simulink model "IFAC20_Random_Exp1_Switched"  (R2019a)
settings: Solver=ode45  StartTime=0.0  StopTime=30  FixedStep=0.05  MaxStep=0.06  RelTol=1e-3  EnableMultiTasking=on
model workspace (MAT data in the model file):
  MCOS : class17 (value not decoded)
values from neighbouring files (symbols this model uses):
  motor_trigger = 1.1    [IFAC20_Experiment2.m]    (also in IFAC20_Experiment3.m = 0.9; IFAC20_Experiment4.m = 0.9)
  wind_trigger = 0.9    [IFAC20_Experiment2.m]    (also in IFAC20_Experiment3.m; IFAC20_Experiment4.m)
undefined symbols (not defined in the file or in its folder): altitude_error, Continuous, IC, quadModel, RPM1, RPM2, RPM3, RPM4, Time
libraries: simulink x9, ctrlSharedLib x4
(part 2 of 2)

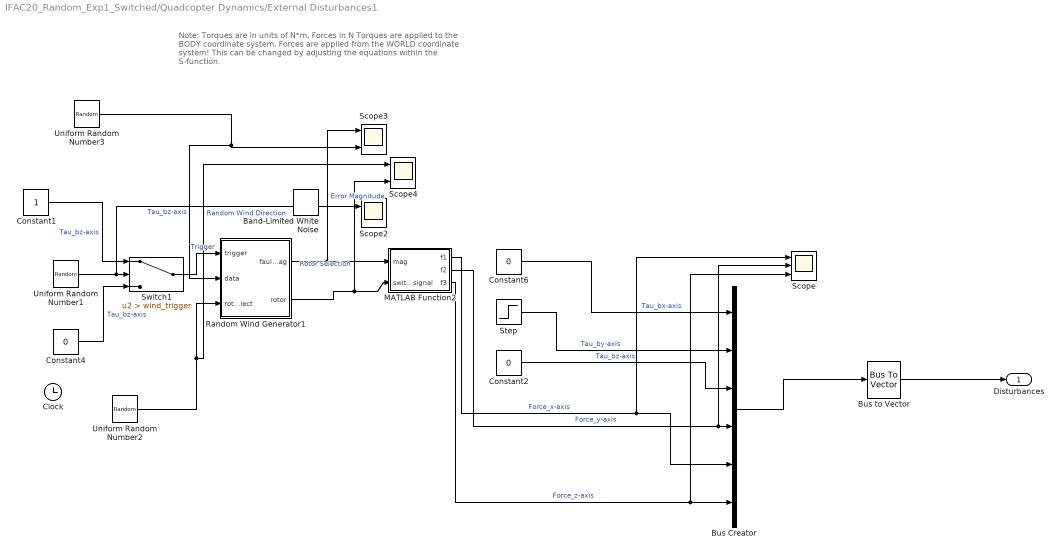
== system IFAC20_Random_Exp1_Switched/Quadcopter Dynamics/External Disturbances1 ==
  note: Note: Torques are in units of N*m, Forces in N
      | Torques are applied to the BODY coordinate system.
      | Forces are applied from the WORLD coordinate system!
      | This can be changed by adjusting the equations within the S-function.
  Band-Limited White Noise : simulink/Sources/Band-Limited White Noise  Cov=[0]  Ts=0.3  seed=[23341]
  Bus Creator : BusCreator  Inputs=6
  Bus to Vector : BusToVector
  Clock : Clock
  Constant1 : Constant
  Constant2 : Constant  Value=0
  Constant4 : Constant  Value=0
  Constant6 : Constant  Value=0
  MATLAB Function2 : MATLAB Function  TreatAsAtomicUnit=on
  Random Wind Generator1 : MATLAB Function  TreatAsAtomicUnit=on
  Scope : Scope  NumInputPorts=3
  Scope2 : Scope  NumInputPorts=2
  Scope3 : Scope  NumInputPorts=2
  Scope4 : Scope  NumInputPorts=2
  Step : Step  After=0  SampleTime=0
  Switch1 : Switch  Criteria=u2 > Threshold  Threshold=wind_trigger
  Uniform Random Number1 : UniformRandomNumber  Minimum=0  Seed=floor(rand(1)*100)  SampleTime=0.1
  Uniform Random Number2 : UniformRandomNumber  Minimum=0.5  Maximum=3.5  Seed=floor(rand(1)*100)  SampleTime=0.1
  Uniform Random Number3 : UniformRandomNumber  Minimum=0  Maximum=10  Seed=floor(rand(1)*100)  SampleTime=0.1
  "Disturbances " : Outport
  wires:
  MATLAB Function2/2(f2) -> Scope/2, Bus Creator/4  "Force_y-axis"
  Random Wind Generator1/1(fault_mag) -> Scope3/1, MATLAB Function2/1(mag)  "Error Magnitude"
  Bus Creator/1 -> Bus to Vector/1
  Constant1/1 -> Switch1/1  "Tau_bz-axis"
  Constant4/1 -> Switch1/3  "Tau_bz-axis"
  Switch1/1 -> Random Wind Generator1/1(trigger)  "Trigger"
  Uniform Random Number3/1 -> Random Wind Generator1/2(data), Scope3/2  "Tau_bz-axis"
  Constant6/1 -> Bus Creator/1  "Tau_bx-axis"
  Bus to Vector/1 -> "Disturbances "/1
  Uniform Random Number1/1 -> Scope2/1, Switch1/2
  Uniform Random Number2/1 -> Scope4/1, Random Wind Generator1/3(rotor_select)  "Random Wind Direction"
  Step/1 -> Bus Creator/2  "Tau_by-axis"
  MATLAB Function2/1(f1) -> Scope/1, Bus Creator/5  "Force_x-axis"
  Random Wind Generator1/2(rotor) -> Scope4/2, MATLAB Function2/2(switch_signal)  "Rotor Selection"
  Constant2/1 -> Bus Creator/3  "Tau_bz-axis"
  MATLAB Function2/3(f3) -> Scope/3, Bus Creator/6  "Force_z-axis"

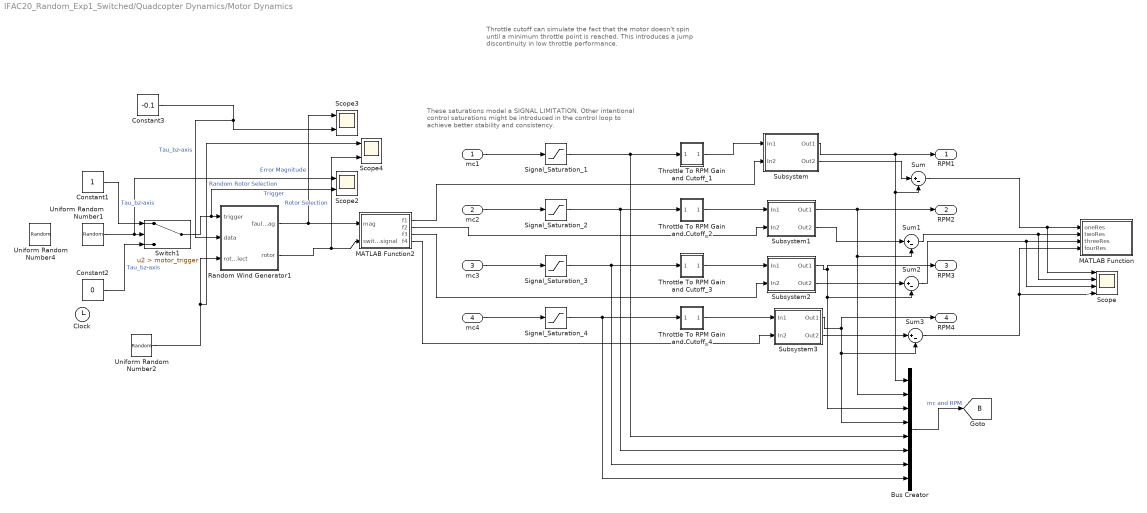
== system IFAC20_Random_Exp1_Switched/Quadcopter Dynamics/Motor Dynamics ==
  note: Throttle cutoff can simulate the fact that the motor doesn't
      | spin until a minimum throttle point is reached. This introduces
      | a jump discontinuity in low throttle performance.
  note: These saturations model a SIGNAL LIMITATION.
      | Other intentional control saturations might be introduced in the
      | control loop to achieve better stability and consistency.
  mc1 : Inport
  mc2 : Inport  Port=2
  mc3 : Inport  Port=3
  mc4 : Inport  Port=4
  Bus Creator : BusCreator  Inputs=8
  Clock : Clock
  Constant1 : Constant
  Constant2 : Constant  Value=0
  Constant3 : Constant  Value=-0.1
  MATLAB Function : MATLAB Function  TreatAsAtomicUnit=on
  MATLAB Function2 : MATLAB Function  TreatAsAtomicUnit=on
  Random Wind Generator1 : MATLAB Function  TreatAsAtomicUnit=on
  Scope : Scope  NumInputPorts=4
  Scope2 : Scope  NumInputPorts=2
  Scope3 : Scope  NumInputPorts=2
  Scope4 : Scope  NumInputPorts=2
  Signal_Saturation_{1..4} (4 alike) : Saturate  UpperLimit=100  LowerLimit=0
  Subsystem : Subsystem
  Subsystem1 : Subsystem
  Subsystem2 : Subsystem
  Subsystem3 : Subsystem
  Sum{,1..3} (4 alike) : Sum  Inputs=|+-
  Switch1 : Switch  Criteria=u2 > Threshold  Threshold=motor_trigger
  Throttle To RPM Gain and Cutoff_1 : Subsystem
  Throttle To RPM Gain and Cutoff_2 : Subsystem
  Throttle To RPM Gain and Cutoff_3 : Subsystem
  Throttle To RPM Gain and Cutoff_4 : Subsystem
  Uniform Random Number1 : UniformRandomNumber  Minimum=0  Seed=floor(rand(1)*100)  SampleTime=0.1
  Uniform Random Number2 : UniformRandomNumber  Minimum=0.5  Maximum=4.5  Seed=floor(rand(1)*100)  SampleTime=0.1
  Uniform Random Number4 : UniformRandomNumber  Minimum=0  Seed=floor(rand(1)*100)  SampleTime=0.1
  RPM1 : Outport
  RPM2 : Outport  Port=2
  RPM3 : Outport  Port=3
  RPM4 : Outport  Port=4
  tag scope: B=global
  wires:
  mc1/1 -> Signal_Saturation_1/1
  mc4/1 -> Signal_Saturation_4/1
  mc2/1 -> Signal_Saturation_2/1
  mc3/1 -> Signal_Saturation_3/1
  Signal_Saturation_1/1 -> Bus Creator/5, Throttle To RPM Gain and Cutoff_1/1(In5)
  Signal_Saturation_2/1 -> Bus Creator/6, Throttle To RPM Gain and Cutoff_2/1(In5)
  Signal_Saturation_3/1 -> Bus Creator/7, Throttle To RPM Gain and Cutoff_3/1(In5)
  Signal_Saturation_4/1 -> Bus Creator/8, Throttle To RPM Gain and Cutoff_4/1(In5)
  Throttle To RPM Gain and Cutoff_4/1(Out5) -> Subsystem3/1(In1)
  Subsystem3/1(Out1) -> RPM4/1, Sum3/2, Bus Creator/4
  Bus Creator/1 -> [B]  "mc and RPM"
  Subsystem/1(Out1) -> Sum/2, Bus Creator/1, RPM1/1
  Throttle To RPM Gain and Cutoff_1/1(Out5) -> Subsystem/1(In1)
  MATLAB Function2/1(f1) -> Subsystem/2(In2)
  Subsystem2/1(Out1) -> Sum2/2, Bus Creator/3, RPM3/1
  Subsystem1/1(Out1) -> Sum1/2, Bus Creator/2, RPM2/1
  Throttle To RPM Gain and Cutoff_2/1(Out5) -> Subsystem1/1(In1)
  Throttle To RPM Gain and Cutoff_3/1(Out5) -> Subsystem2/1(In1)
  MATLAB Function2/3(f3) -> Subsystem2/2(In2)
  MATLAB Function2/4(f4) -> Subsystem3/2(In2)
  MATLAB Function2/2(f2) -> Subsystem1/2(In2)
  Subsystem/2(Out2) -> Sum/1
  Sum/1 -> Scope/1, MATLAB Function/1(oneRes)
  Subsystem3/2(Out2) -> Sum3/1
  Subsystem2/2(Out2) -> Sum2/1
  Subsystem1/2(Out2) -> Sum1/1
  Sum3/1 -> Scope/4, MATLAB Function/4(fourRes)
  Sum2/1 -> Scope/3, MATLAB Function/3(threeRes)
  Sum1/1 -> Scope/2, MATLAB Function/2(twoRes)
  Random Wind Generator1/1(fault_mag) -> Scope3/1, MATLAB Function2/1(mag)  "Error Magnitude"
  Constant2/1 -> Switch1/3  "Tau_bz-axis"
  Uniform Random Number2/1 -> Scope4/1, Random Wind Generator1/3(rotor_select)  "Random Rotor Selection"
  Random Wind Generator1/2(rotor) -> Scope4/2, MATLAB Function2/2(switch_signal)  "Rotor Selection"
  Uniform Random Number1/1 -> Scope2/1, Switch1/2
  Constant1/1 -> Switch1/1  "Tau_bz-axis"
  Constant3/1 -> Random Wind Generator1/2(data), Scope3/2  "Tau_bz-axis"
  Switch1/1 -> Scope2/2, Random Wind Generator1/1(trigger)  "Trigger"

== system IFAC20_Random_Exp1_Switched/Quadcopter Dynamics/Motor Dynamics/Subsystem ==
  note: kalman filter
  note: Multiplicitive Fault
  In1 : Inport
  In2 : Inport  Port=2
  Kalman Filter : ctrlSharedLib/Kalman Filter  TimeDomain=Continuous-Time  UseCurrentEstimator=on  ModelSource=Individual A, B, C, D matrices  ModelSourceVariable=quadcopterDynamicsSFunction  A=-1/quadModel.T  B=1  C=1/quadModel.T  D=0  NumberOfStates=1  NumberOfInputs=1  NumberOfOutputs=1  InitialEstimateSource=Dialog  X0=0  P0=10  UseK=off  UseGH=off  NumberOfProcessNoiseInputs=1  G=1  TimeInvariantG=on  H=0  TimeInvariantH=on  Q=0.05  TimeInvariantQ=on  R=1  TimeInvariantR=on  N=0  TimeInvariantN=on  AddInputPort=on  AddEnablePort=off  OutputEstimatedY=on  OutputP=off  Ts=-1
      settings: SourceProductBaseCode=CT
  MATLAB Function : MATLAB Function  TreatAsAtomicUnit=on
  Motor_Dynamics_1 : StateSpace  A=-1/quadModel.T  C=1/quadModel.T  D=0  InitialCondition=IC.w1*quadModel.T
  Out1 : Outport
  Out2 : Outport  Port=2
  wires:
  In1/1 -> Kalman Filter/1, Motor_Dynamics_1/1
  MATLAB Function/1(rotor_speed) -> Out1/1, Kalman Filter/2
  In2/1 -> MATLAB Function/1(fault)
  Motor_Dynamics_1/1 -> MATLAB Function/2(nominal_model_input)
  Kalman Filter/2 -> Out2/1

== system IFAC20_Random_Exp1_Switched/Quadcopter Dynamics/Motor Dynamics/Subsystem1 ==
  In1 : Inport
  In2 : Inport  Port=2
  Kalman Filter : ctrlSharedLib/Kalman Filter  TimeDomain=Continuous-Time  UseCurrentEstimator=on  ModelSource=Individual A, B, C, D matrices  ModelSourceVariable=quadcopterDynamicsSFunction  A=-1/quadModel.T  B=1  C=1/quadModel.T  D=0  NumberOfStates=1  NumberOfInputs=1  NumberOfOutputs=1  InitialEstimateSource=Dialog  X0=0  P0=10  UseK=off  UseGH=off  NumberOfProcessNoiseInputs=1  G=1  TimeInvariantG=on  H=0  TimeInvariantH=on  Q=0.05  TimeInvariantQ=on  R=1  TimeInvariantR=on  N=0  TimeInvariantN=on  AddInputPort=on  AddEnablePort=off  OutputEstimatedY=on  OutputP=off  Ts=-1
      settings: SourceProductBaseCode=CT
  MATLAB Function : MATLAB Function  TreatAsAtomicUnit=on
  "Motor_Dynamics_2 " : StateSpace  A=-1/quadModel.T  C=1/quadModel.T  D=0  InitialCondition=IC.w1*quadModel.T
  Out1 : Outport
  Out2 : Outport  Port=2
  wires:
  In1/1 -> "Motor_Dynamics_2 "/1, Kalman Filter/1
  MATLAB Function/1(rotor_speed) -> Kalman Filter/2, Out1/1
  In2/1 -> MATLAB Function/1(fault)
  "Motor_Dynamics_2 "/1 -> MATLAB Function/2(nominal_modal_input)
  Kalman Filter/2 -> Out2/1

== system IFAC20_Random_Exp1_Switched/Quadcopter Dynamics/Motor Dynamics/Subsystem2 ==
  In1 : Inport
  In2 : Inport  Port=2
  Kalman Filter : ctrlSharedLib/Kalman Filter  TimeDomain=Continuous-Time  UseCurrentEstimator=on  ModelSource=Individual A, B, C, D matrices  ModelSourceVariable=quadcopterDynamicsSFunction  A=-1/quadModel.T  B=1  C=1/quadModel.T  D=0  NumberOfStates=1  NumberOfInputs=1  NumberOfOutputs=1  InitialEstimateSource=Dialog  X0=0  P0=10  UseK=off  UseGH=off  NumberOfProcessNoiseInputs=1  G=1  TimeInvariantG=on  H=0  TimeInvariantH=on  Q=0.05  TimeInvariantQ=on  R=1  TimeInvariantR=on  N=0  TimeInvariantN=on  AddInputPort=on  AddEnablePort=off  OutputEstimatedY=on  OutputP=off  Ts=-1
      settings: SourceProductBaseCode=CT
  MATLAB Function : MATLAB Function  TreatAsAtomicUnit=on
  "Motor_Dynamics_3 " : StateSpace  A=-1/quadModel.T  C=1/quadModel.T  D=0  InitialCondition=IC.w1*quadModel.T
  Out1 : Outport
  Out2 : Outport  Port=2
  wires:
  In1/1 -> "Motor_Dynamics_3 "/1, Kalman Filter/1
  MATLAB Function/1(rotor_speed) -> Kalman Filter/2, Out1/1
  In2/1 -> MATLAB Function/1(fault)
  "Motor_Dynamics_3 "/1 -> MATLAB Function/2(nominal_modal_input)
  Kalman Filter/2 -> Out2/1

== system IFAC20_Random_Exp1_Switched/Quadcopter Dynamics/Motor Dynamics/Subsystem3 ==
  In1 : Inport
  In2 : Inport  Port=2
  Kalman Filter : ctrlSharedLib/Kalman Filter  TimeDomain=Continuous-Time  UseCurrentEstimator=on  ModelSource=Individual A, B, C, D matrices  ModelSourceVariable=quadcopterDynamicsSFunction  A=-1/quadModel.T  B=1  C=1/quadModel.T  D=0  NumberOfStates=1  NumberOfInputs=1  NumberOfOutputs=1  InitialEstimateSource=Dialog  X0=0  P0=10  UseK=off  UseGH=off  NumberOfProcessNoiseInputs=1  G=1  TimeInvariantG=on  H=0  TimeInvariantH=on  Q=0.05  TimeInvariantQ=on  R=1  TimeInvariantR=on  N=0  TimeInvariantN=on  AddInputPort=on  AddEnablePort=off  OutputEstimatedY=on  OutputP=off  Ts=-1
      settings: SourceProductBaseCode=CT
  MATLAB Function : MATLAB Function  TreatAsAtomicUnit=on
  "Motor_Dynamics_4 " : StateSpace  A=-1/quadModel.T  C=1/quadModel.T  D=0  InitialCondition=IC.w1*quadModel.T
  Out1 : Outport
  Out2 : Outport  Port=2
  wires:
  In1/1 -> Kalman Filter/1, "Motor_Dynamics_4 "/1
  MATLAB Function/1(rotor_speed) -> Kalman Filter/2, Out1/1
  In2/1 -> MATLAB Function/1(fault)
  "Motor_Dynamics_4 "/1 -> MATLAB Function/2(nominal_modal_input)
  Kalman Filter/2 -> Out2/1

== system IFAC20_Random_Exp1_Switched/Quadcopter Dynamics/Motor Dynamics/Throttle To RPM Gain and Cutoff_1 ==
  note: minThr should be a quad.mat value
  note: This gain should be a quad.mat value
  note: This constant should be a quad.mat value
  note: Output equals linearly scaled RPM
      | for given throttle input if throttle input >=Throttle Cuttoff (minThr)
      | else output is zero.
  In5 : Inport
  Constant : Constant  Value=quadModel.b
  Gain : Gain  Gain=quadModel.cr
  Minimum Throttle Cutoff : simulink/Logic and Bit Operations/Compare To Constant  relop=>=  const=quadModel.minThr  OutDataTypeStr=uint8
  Product : Product
  Sum1 : Sum  Inputs=++|
  Out5 : Outport
  wires:
  Minimum Throttle Cutoff/1 -> Product/2
  Product/1 -> Out5/1
  In5/1 -> Gain/1, Minimum Throttle Cutoff/1
  Gain/1 -> Sum1/2
  Sum1/1 -> Product/1
  Constant/1 -> Sum1/1

== system IFAC20_Random_Exp1_Switched/Quadcopter Dynamics/Motor Dynamics/Throttle To RPM Gain and Cutoff_2 ==
  note: minThr should be a quad.mat value
  note: This gain should be a quad.mat value
  note: This constant should be a quad.mat value
  note: Output equals linearly scaled RPM
      | for given throttle input if throttle input >=Throttle Cuttoff (minThr)
      | else output is zero.
  In5 : Inport
  Constant : Constant  Value=quadModel.b
  Gain : Gain  Gain=quadModel.cr
  Minimum Throttle Cutoff : simulink/Logic and Bit Operations/Compare To Constant  relop=>=  const=quadModel.minThr  OutDataTypeStr=uint8
  Product : Product
  Sum1 : Sum  Inputs=++|
  Out5 : Outport
  wires:
  Minimum Throttle Cutoff/1 -> Product/2
  Product/1 -> Out5/1
  In5/1 -> Gain/1, Minimum Throttle Cutoff/1
  Gain/1 -> Sum1/2
  Sum1/1 -> Product/1
  Constant/1 -> Sum1/1

== system IFAC20_Random_Exp1_Switched/Quadcopter Dynamics/Motor Dynamics/Throttle To RPM Gain and Cutoff_3 ==
  note: minThr should be a quad.mat value
  note: This gain should be a quad.mat value
  note: This constant should be a quad.mat value
  note: Output equals linearly scaled RPM
      | for given throttle input if throttle input >=Throttle Cuttoff (minThr)
      | else output is zero.
  In5 : Inport
  Constant : Constant  Value=quadModel.b
  Gain : Gain  Gain=quadModel.cr
  Minimum Throttle Cutoff : simulink/Logic and Bit Operations/Compare To Constant  relop=>=  const=quadModel.minThr  OutDataTypeStr=uint8
  Product : Product
  Sum1 : Sum  Inputs=++|
  Out5 : Outport
  wires:
  Minimum Throttle Cutoff/1 -> Product/2
  Product/1 -> Out5/1
  In5/1 -> Gain/1, Minimum Throttle Cutoff/1
  Gain/1 -> Sum1/2
  Sum1/1 -> Product/1
  Constant/1 -> Sum1/1

== system IFAC20_Random_Exp1_Switched/Quadcopter Dynamics/Motor Dynamics/Throttle To RPM Gain and Cutoff_4 ==
  note: minThr should be a quad.mat value
  note: This gain should be a quad.mat value
  note: This constant should be a quad.mat value
  note: Output equals linearly scaled RPM
      | for given throttle input if throttle input >=Throttle Cuttoff (minThr)
      | else output is zero.
  In5 : Inport
  Constant : Constant  Value=quadModel.b
  Gain : Gain  Gain=quadModel.cr
  Minimum Throttle Cutoff : simulink/Logic and Bit Operations/Compare To Constant  relop=>=  const=quadModel.minThr  OutDataTypeStr=uint8
  Product : Product
  Sum1 : Sum  Inputs=++|
  Out5 : Outport
  wires:
  Minimum Throttle Cutoff/1 -> Product/2
  Product/1 -> Out5/1
  In5/1 -> Gain/1, Minimum Throttle Cutoff/1
  Gain/1 -> Sum1/2
  Sum1/1 -> Product/1
  Constant/1 -> Sum1/1

== matlab function IFAC20_Random_Exp1_Switched/Quadcopter Dynamics/Motor Dynamics/Subsystem/MATLAB Function ==
  data: fault input; nominal_model_input input; rotor_speed output
function rotor_speed = fcn(fault, nominal_model_input)

rotor_speed =(nominal_model_input* (1-fault));

end

== matlab function IFAC20_Random_Exp1_Switched/Attitude Controller/blending  ==
  settings: updateMethod=DISCRETE
  data: control_signal output; trigger input; fault_controller input; nominal_controller input; portion output
function [control_signal ,portion] = blending(trigger, fault_controller, nominal_controller)


portion = trigger;
fault_part = (fault_controller * portion);
nominal_portion = 1-portion;
nominal_part = nominal_controller * nominal_portion;
control_signal = fault_part + nominal_part;

end

== matlab function IFAC20_Random_Exp1_Switched/Quadcopter Dynamics/Motor Dynamics/Subsystem1/MATLAB Function ==
  data: fault input; nominal_modal_input input; rotor_speed output
function rotor_speed = fcn(  fault, nominal_modal_input)


rotor_speed =  (nominal_modal_input* (1-fault));

end

== matlab function IFAC20_Random_Exp1_Switched/Position Controller/MATLAB Function ==
  settings: updateMethod=DISCRETE
  data: y_error input; x_error input; max_error_signal data_store_memory; count data_store_memory; time input; prevTime data_store_memory
function fcn(y_error,x_error,time)
global prevTime;
global max_error_signal;
global count;
%if(abs(y_error) + abs(x_error) > max_error_signal)
if(prevTime+0.1 < time)
    max_error_signal = max_error_signal + abs(y_error) + abs(x_error);
    count =count +1;
    %disp(count);
    prevTime = time;
end
end

== matlab function IFAC20_Random_Exp1_Switched/Quadcopter Dynamics/Motor Dynamics/Subsystem2/MATLAB Function ==
  data: fault input; nominal_modal_input input; rotor_speed output
function rotor_speed = fcn(  fault, nominal_modal_input)


rotor_speed =  (nominal_modal_input* (1-fault));

end

== matlab function IFAC20_Random_Exp1_Switched/Quadcopter Dynamics/Motor Dynamics/Subsystem3/MATLAB Function ==
  data: fault input; nominal_modal_input input; rotor_speed output
function rotor_speed = fcn(  fault, nominal_modal_input)


rotor_speed =  (nominal_modal_input* (1-fault));

end

== matlab function IFAC20_Random_Exp1_Switched/Attitude Controller/blending 1 ==
  settings: updateMethod=DISCRETE
  data: control_signal output; trigger input; fault_controller input; nominal_controller input; portion output
function [control_signal,portion] = blending(trigger,fault_controller, nominal_controller)


portion = trigger;
fault_part = (fault_controller * portion);
nominal_portion = 1-portion;
nominal_part = nominal_controller * nominal_portion;
control_signal = fault_part + nominal_part;

end

== matlab function IFAC20_Random_Exp1_Switched/Attitude Controller/blending 2 ==
  data: control_signal output; portion input; fault_controller input; nominal_controller input
function control_signal = blending(portion , fault_controller, nominal_controller)

fault_part = (fault_controller * portion);
nominal_portion = 1-portion;
nominal_part = nominal_controller * nominal_portion;
control_signal = fault_part + nominal_part;

end

== matlab function IFAC20_Random_Exp1_Switched/Quadcopter Dynamics/External Disturbances1/MATLAB Function2 ==
  data: mag input; f1 output; switch_signal input; f2 output; f3 output
function [f1,f2,f3] = fcn(mag , switch_signal)

f1 = 0;
f2 = 0;
f3 = 0;

if switch_signal == 1
    f1 = mag;
elseif switch_signal ==2
    f2 = mag;
elseif switch_signal ==3
    f3 = mag;
end

== matlab function IFAC20_Random_Exp1_Switched/Position Controller/MATLAB Function1 ==
  settings: updateMethod=DISCRETE
  data: alt_diff input; y output; altitude_error data_store_memory; time input; PrevTime2 data_store_memory
function y = fcn(alt_diff, time)
global altitude_error;
global PrevTime2;

if(PrevTime2+0.1 < time)
    altitude_error = altitude_error + abs(alt_diff);

    y = altitude_error;
    PrevTime2 = time;
else
    y = altitude_error;
end

== matlab function IFAC20_Random_Exp1_Switched/Quadcopter Dynamics/Motor Dynamics/MATLAB Function ==
  settings: updateMethod=DISCRETE
  data: oneRes input; twoRes input; threeRes input; fourRes input; fault_est data_store_memory
function fcn(oneRes, twoRes, threeRes, fourRes)
global fault_est;
maxRes = max([oneRes twoRes threeRes fourRes]);
%threshold in rpm
threshold = 50;

if(maxRes > threshold)
    fault_est = 1;
else
    fault_est = 0;
end

== matlab function IFAC20_Random_Exp1_Switched/Position Controller/Position Randomization ==
  settings: updateMethod=DISCRETE
  data: Xd input; Xr input; Phi output; Theta output; Yd input; Yr input
function [Phi, Theta] = fcn(Xd, Xr, Yd, Yr)

pos = [Xd, Xr, Yd, Yr];
current_error = pdist(pos,'euclidean');
disp(current_error);
random = false;
if( random)
    
    blend = rand();
    %blend =0;
    Phi = blend;
    Theta= blend;
else
    %blend = rand();
    blend =0;
    Phi = blend;
    Theta= blend;
end

== matlab function IFAC20_Random_Exp1_Switched/Position Controller/blending 1 ==
  data: Phi_cmd output; portion input; fault_controller input; nominal_controller input
function Phi_cmd = blending(portion , fault_controller, nominal_controller)

fault_part = (fault_controller * portion);
nominal_portion = 1-portion;
nominal_part = nominal_controller * nominal_portion;
Phi_cmd = fault_part + nominal_part;

end

== matlab function IFAC20_Random_Exp1_Switched/Position Controller/blending 2 ==
  data: The_cmd output; portion input; fault_controller input; nominal_controller input
function The_cmd = blending(portion , fault_controller, nominal_controller)

fault_part = (fault_controller * portion);
nominal_portion = 1-portion;
nominal_part = nominal_controller * nominal_portion;
The_cmd = fault_part + nominal_part;

end

== matlab function IFAC20_Random_Exp1_Switched/Quadcopter Dynamics/External Disturbances1/Random Wind Generator1 ==
  settings: updateMethod=DISCRETE
  data: fault_mag output; rotor output; trigger input; data input; rotor_select input
function [fault_mag,rotor] = fcn( trigger, data, rotor_select)


if(trigger == 1)
    
    fault_mag = data;
    rotor = round(rotor_select);
else
    fault_mag = 0;
    rotor = 0;
end

== matlab function IFAC20_Random_Exp1_Switched/Quadcopter Dynamics/Motor Dynamics/MATLAB Function2 ==
  data: mag input; f1 output; switch_signal input; f2 output; f3 output; f4 output
function [f1,f2,f3,f4] = fcn(mag , switch_signal)

f1 = 0;
f2 = 0;
f3 = 0;
f4 = 0;

if switch_signal == 1
    f1 = mag;
elseif switch_signal ==2
    f2 = mag;
elseif switch_signal ==3
    f3 = mag;
elseif switch_signal ==4
    f4 = mag;
end

== matlab function IFAC20_Random_Exp1_Switched/Quadcopter Dynamics/Motor Dynamics/Random Wind Generator1 ==
  settings: updateMethod=DISCRETE
  data: fault_mag output; rotor output; trigger input; data input; rotor_select input
function [fault_mag,rotor] = fcn( trigger, data, rotor_select)


    if(trigger == 1)

        fault_mag = data;
        rotor = round(rotor_select);
        
    else
        fault_mag = 0;
        rotor = 0;
    end
